simulink model "simulink_rohrs"  (R2015b)
settings: Solver=VariableStepAuto  StartTime=0.0  StopTime=14  RelTol=1e-3
values from neighbouring files (symbols this model uses):
  am = -3    [Matlab_uppg3.m]
  ap = -1    [Matlab_uppg3.m]
  Gamma = eye(2*n).*100    [Matlab_exam.m]    (also in Matlab_uppg3.m = eye(2).*3)
  km = 3    [Matlab_uppg3.m]
  kp = 2    [Matlab_uppg3.m]
  sys_r = ss(P_rohr)    [Matlab_uppg3.m]
  theta_init = zeros(n+m+1,1)    [Matlab_uppg2.m]    (also in Matlab_uppg3.m = zeros(2,1))
  xm_init = 0    [Matlab_uppg3.m]
  xp_init = 0    [Matlab_uppg3.m]
libraries: simulink x1
settings Model: Creator=Albin  LastModifiedBy=Albin

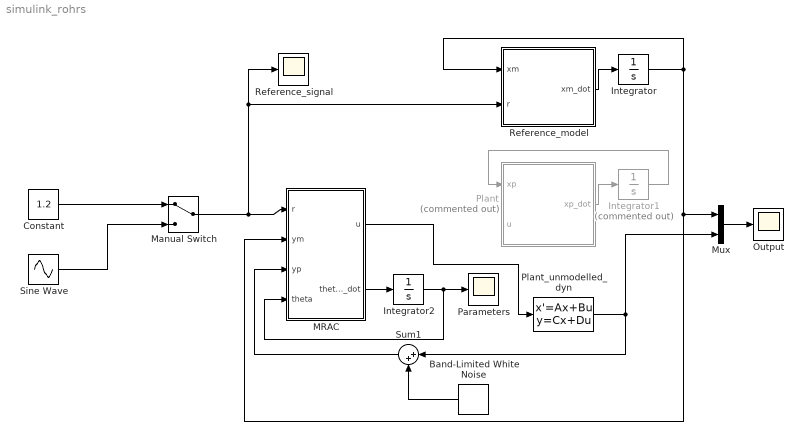
== system simulink_rohrs ==
  Band-Limited White Noise : simulink/Sources/Band-Limited White Noise  Cov=[0.01]  Ts=0.1  seed=[23341]
  Constant : Constant  Value=1.2
  Integrator : Integrator  InitialCondition=xm_init
  Integrator1 : Integrator  Commented=on  InitialCondition=xp_init
  Integrator2 : Integrator  InitialCondition=theta_init
  MRAC : MATLAB Function  TreatAsAtomicUnit=on
  Manual Switch : ManualSwitch
  Mux : Mux  Inputs=2
  Output : Scope
  Parameters : Scope
  Plant : MATLAB Function  Commented=on  TreatAsAtomicUnit=on
  "Plant_unmodelled_dyn " : StateSpace  A=sys_r.A  B=sys_r.B  C=sys_r.C  D=sys_r.D  X0=0
  Reference_model : MATLAB Function  TreatAsAtomicUnit=on
  Reference_signal : Scope
  Sine Wave : Sin  SampleTime=0
  Sum1 : Sum  Inputs=|++
  wires:
  Reference_model/1(xm_dot) -> Integrator/1
  Plant/1(xp_dot) -> Integrator1/1
  MRAC/2(theta_dot) -> Integrator2/1
  Integrator2/1 -> Parameters/1, MRAC/4(theta)
  Integrator/1 -> Mux/1, MRAC/2(ym), Reference_model/1(xm)
  Integrator1/1 -> Plant/1(xp)
  Manual Switch/1 -> Reference_signal/1, Reference_model/2(r), MRAC/1(r)
  Constant/1 -> Manual Switch/1
  Mux/1 -> Output/1
  MRAC/1(u) -> "Plant_unmodelled_dyn "/1
  "Plant_unmodelled_dyn "/1 -> Sum1/1, Mux/2
  Sine Wave/1 -> Manual Switch/2
  Sum1/1 -> MRAC/3(yp)
  Band-Limited White Noise/1 -> Sum1/2

== matlab function simulink_rohrs/Reference_model ==
  data: xm input; xm_dot output; r input; am parameter; km parameter
function xm_dot  = fcn(xm,r,am,km)
%#codegen
xm_dot = am*xm + km*r;

== matlab function simulink_rohrs/Plant ==
  data: xp input; xp_dot output; u input; ap parameter; kp parameter
function xp_dot  = fcn(xp,u,ap,kp)
%#codegen

xp_dot = ap*xp + kp*u;      % Simplified plant

xp_dot =

== matlab function simulink_rohrs/MRAC ==
  data: r input; ym input; u output; theta_dot output; yp input; theta input; kp parameter; Gamma parameter
function [u,theta_dot] = fcn(r,ym,yp,theta,kp,Gamma)
%#codegen
error = yp-ym;

phi = [r,yp]';

theta_dot = -sign(kp)*Gamma*error*phi;

u = theta'*phi;
